simulink model "untitled"  (R2019b)
settings: Solver=VariableStepAuto  StartTime=0.0  StopTime=10.0  RelTol=1e-3
libraries: commutil2 x2, dspquant2 x2, dsparch4 x1, dspsigops x1
settings Model: Creator=DELL  LastModifiedBy=DELL

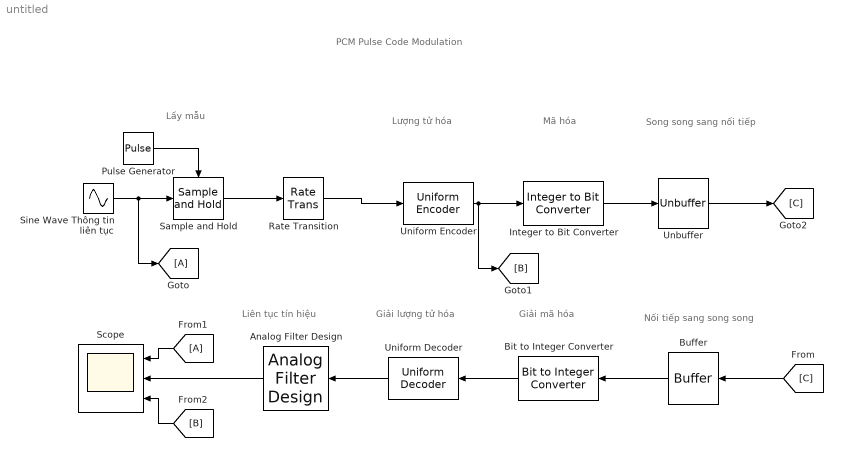
== system untitled ==
  note: Lấy mẫu
  note: PCM Pulse Code Modulation
  note: Lượng tử hóa
  note: Mã hóa
  note: Song song
      | sang nối tiếp
  note: Nối tiếp
      | sang song song
  note: Giải mã hóa
  note: Giải lượng tử hóa
  note: Liên tục tín hiệu
  Analog Filter Design : dsparch4/Analog Filter Design  method=Butterworth  filttype=Lowpass  N=12  Wlo=2*pi*4000  Whi=80  Rp=2  Rs=40
  Bit to Integer Converter : commutil2/Bit to Integer Converter  nbits=3  bitOrder=MSB first  signedOutputValues=Unsigned  outDtype=Inherit via internal rule  outDtypeSigned=Inherit via internal rule
      settings: SourceProductName=Communications Toolbox
  Buffer : Buffer  N=3  OutputFrames=off
  Integer to Bit Converter : commutil2/Integer to Bit Converter  nbits=3  signedInputValues=Unsigned  bitOrder=MSB first  outDtype=Inherit via internal rule
      settings: SourceProductName=Communications Toolbox
  Pulse Generator : DiscretePulseGenerator  PulseType=Time based  Period=1/8000  PulseWidth=5
  Rate Transition : RateTransition  OutPortSampleTime=1/8000
  Sample and Hold : dspsigops/Sample and Hold  trig=Rising edge  initCond=0  latchinput=off
  Scope : Scope  NumInputPorts=3
  Sine Wave Thông tin liên tục : Sin  Frequency=2*pi*3000  SampleTime=1/100000
  Unbuffer : Unbuffer
  Uniform Decoder : dspquant2/Uniform Decoder  peak=1  bits=3  overflowMode=Saturate  otype=Double
      settings: SourceProductName=DSP System Toolbox  SourceProductBaseCode=DS
  Uniform Encoder : dspquant2/Uniform Encoder  peak=1  bits=3  otype=Unsigned integer
      settings: SourceProductName=DSP System Toolbox
  wires:
  Sine Wave Thông tin liên tục/1 -> [A], Sample and Hold/1
  Pulse Generator/1 -> Sample and Hold/Trigger
  Uniform Encoder/1 -> [B], Integer to Bit Converter/1
  Integer to Bit Converter/1 -> Unbuffer/1
  Unbuffer/1 -> [C]
  [C] -> Buffer/1
  Bit to Integer Converter/1 -> Uniform Decoder/1
  Buffer/1 -> Bit to Integer Converter/1
  Uniform Decoder/1 -> Analog Filter Design/1
  Analog Filter Design/1 -> Scope/2
  [A] -> Scope/1
  [B] -> Scope/3
  Rate Transition/1 -> Uniform Encoder/1
  Sample and Hold/1 -> Rate Transition/1
